simulink model "Parabolic_alpha_sim"  (R2017a)
settings: Solver=FixedStepAuto  StartTime=0.0  StopTime=4  FixedStep=2e-4  RelTol=1e-3
values from neighbouring files (symbols this model uses):
  b = 2.8956    [Aerosonde_coeff.m]    (also in coeff_Aerosonde.m)
  c = 0.18994    [Aerosonde_coeff.m]    (also in coeff_Aerosonde.m)
  C_De = 0    [Aerosonde_coeff.m]    (also in coeff_Aerosonde.m)
  C_Dl_quad = 0.05*2    (= 0.1)    [coeff_quad.m]    (also in init_quad.m = 0.05)
  C_Dq = 0    [Aerosonde_coeff.m]    (also in coeff_Aerosonde.m)
  C_Dq_quad = 0.5    [coeff_quad.m]    (also in init_quad.m)
  C_Le = -0.36    [Aerosonde_coeff.m]    (also in coeff_Aerosonde.m)
  C_Lq = 0    [Aerosonde_coeff.m]    (also in coeff_Aerosonde.m)
  C_m0 = -0.02338    [Aerosonde_coeff.m]    (also in coeff_Aerosonde.m)
  C_ma = -0.38    [Aerosonde_coeff.m]    (also in coeff_Aerosonde.m)
  C_me = -0.5    [Aerosonde_coeff.m]    (also in coeff_Aerosonde.m)
  C_mq = -3.6    [Aerosonde_coeff.m]    (also in coeff_Aerosonde.m)
  d_m_quad = 0.15    [coeff_quad.m]    (also in init_quad.m)
  g = 9.81    [coeff_quad.m]    (also in init_quad.m)
  J_quad = 0.2    [coeff_quad.m]    (also in init_quad.m)
  m_quad = 2.5    [coeff_quad.m]    (also in init_quad.m)
  max_sum_force = 80    [coeff_quad.m]    (also in init_quad.m = 100)
  quad_init_theta = -20*deg2rad    [init__Aerosonde_and_quad.m]    (also in init_quad.m = -0.349065850399)
  quad_init_vx = 15    [init__Aerosonde_and_quad.m]    (also in init_quad.m)
  quad_init_vz = 0    [init__Aerosonde_and_quad.m]    (also in init_quad.m)
  quad_init_x = -8    [init__Aerosonde_and_quad.m]    (also in init_quad.m)
  quad_init_z = -dist_z-2    [init__Aerosonde_and_quad.m]    (also in init_quad.m = -20)
  rho = 1.2682    [Aerosonde_coeff.m]    (also in coeff_Aerosonde.m)
undefined symbols (not defined in the file or in its folder): Newton, Raphson
libraries: simulink_extras x8, aerolibasang x3, shared3dof x1, aerolibadyn x1
settings Model: Creator=jljoberg  LastModifiedBy=jljoberg

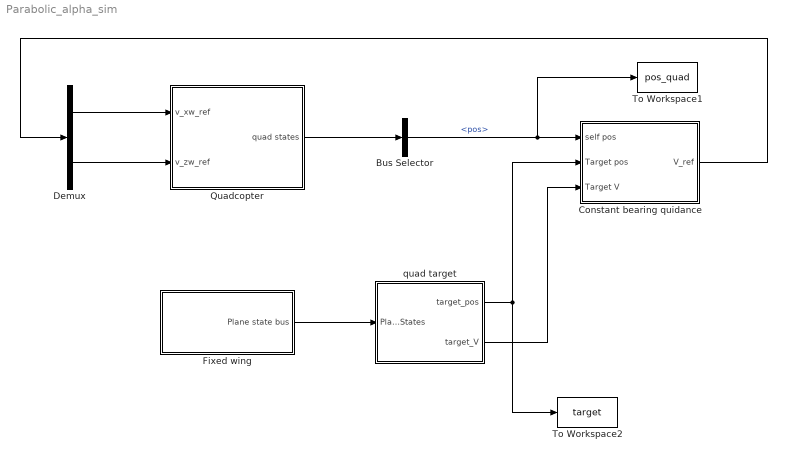
== system Parabolic_alpha_sim ==
  Bus Selector : BusSelector  OutputSignals=pos
  Constant bearing quidance : Subsystem
  Demux : Demux  Outputs=2
  Fixed wing : Subsystem
  Quadcopter : Subsystem
  To Workspace1 : ToWorkspace  VariableName=pos_quad  SaveFormat=Timeseries  SampleTime=-1
  To Workspace2 : ToWorkspace  VariableName=target  SaveFormat=Timeseries  SampleTime=-1
  quad target : Subsystem
  wires:
  Fixed wing/1(Plane state bus) -> quad target/1(Plane States)
  quad target/1(target_pos) -> Constant bearing quidance/2(Target pos), To Workspace2/1
  quad target/2(target_V) -> Constant bearing quidance/3(Target V)
  Quadcopter/1(quad states) -> Bus Selector/1
  Bus Selector/1 -> To Workspace1/1, Constant bearing quidance/1(self pos)  "<pos>"
  Constant bearing quidance/1(V_ref) -> Demux/1
  Demux/2 -> Quadcopter/2(v_zw_ref)
  Demux/1 -> Quadcopter/1(v_xw_ref)

== system Parabolic_alpha_sim/Constant bearing quidance ==
  self pos : Inport
  Target pos : Inport  Port=2
  Target V : Inport  Port=3
  CBG : MATLAB Function  TreatAsAtomicUnit=on
  V_ref : Outport
  wires:
  self pos/1 -> CBG/1(p)
  Target pos/1 -> CBG/2(p_t)
  Target V/1 -> CBG/3(V_t)
  CBG/1(V_ref) -> V_ref/1

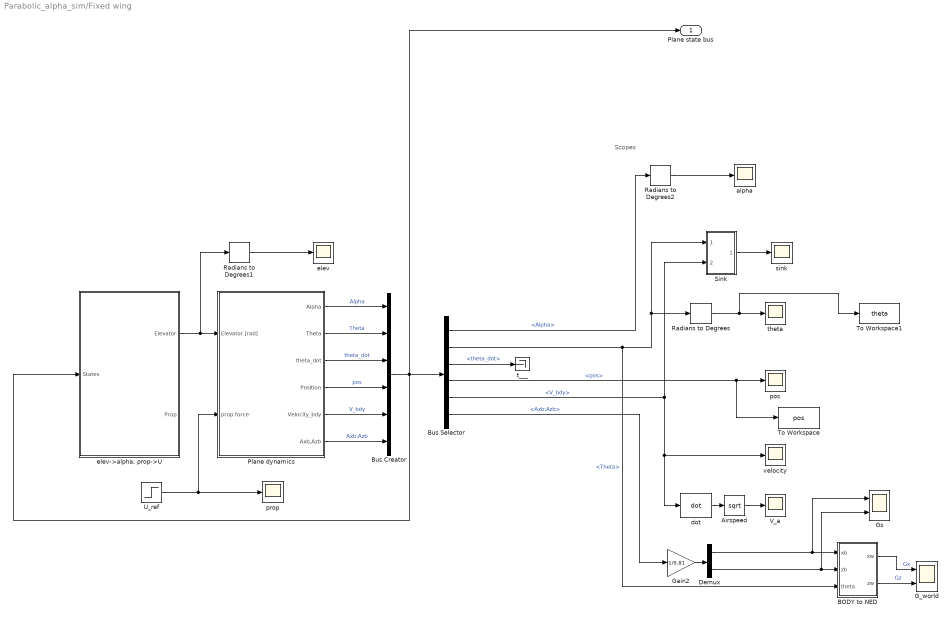
== system Parabolic_alpha_sim/Fixed wing ==
  note: Scopes
  Airspeed : Sqrt  AlgorithmType=Newton-Raphson  SaturateOnIntegerOverflow=on
  BODY to NED : Subsystem
  Bus Creator : BusCreator  Inputs=6
  Bus Selector : BusSelector  OutputSignals=Alpha,Theta,theta_dot,pos,V_bdy,Axb;Azb
  Demux : Demux  Outputs=2
  G_world : Scope  NumInputPorts=2
  Gain2 : Gain  Gain=1/9.81
  Gs : Scope  NumInputPorts=2
  Plane dynamics : Subsystem
  Radians to Degrees : simulink_extras/Transformations/Radians to Degrees
  Radians to Degrees1 : simulink_extras/Transformations/Radians to Degrees
  Radians to Degrees2 : simulink_extras/Transformations/Radians to Degrees
  Sink : Subsystem
  To Workspace : ToWorkspace  VariableName=pos  SaveFormat=Timeseries  SampleTime=-1
  To Workspace1 : ToWorkspace  VariableName=theta  SaveFormat=Timeseries  SampleTime=-1
  U_ref : Step  Time=10.5  After=0  SampleTime=0
  V_a : Scope
  alpha : Scope
  dot : aerolibasang/Incidence  & Airspeed/dot
      settings: SourceProductName=Aerospace Blockset  SourceProductBaseCode=AE
  elev : Scope
  elev->alpha; prop->U : Subsystem  VariantControl=Variant
  pos : Scope
  prop : Scope
  sink : Scope
  t___ : Terminator
  theta : Scope
  velocity : Scope
  Plane state bus : Outport
  wires:
  Plane dynamics/3(theta_dot) -> Bus Creator/3  "theta_dot"
  Plane dynamics/2(Theta) -> Bus Creator/2  "Theta"
  Plane dynamics/1(Alpha) -> Bus Creator/1  "Alpha"
  Airspeed/1 -> V_a/1
  Bus Selector/3 -> t___/1  "<theta_dot>"
  Bus Selector/4 -> To Workspace/1, pos/1  "<pos>"
  Bus Selector/5 -> dot/1, velocity/1, Sink/2(v_bdy)  "<V_bdy>"
  Bus Selector/2 -> BODY to NED/3(theta), Radians to Degrees/1, Sink/1(theta)  "<Theta>"
  Radians to Degrees/1 -> To Workspace1/1, theta/1
  Sink/1(sink) -> sink/1
  Bus Selector/1 -> Radians to Degrees2/1  "<Alpha>"
  Plane dynamics/6(Axb,Azb) -> Bus Creator/6  "Axb;Azb"
  dot/1 -> Airspeed/1
  Plane dynamics/5(Velocity_bdy) -> Bus Creator/5  "V_bdy"
  Plane dynamics/4(Position) -> Bus Creator/4  "pos"
  Demux/1 -> BODY to NED/1(xb), Gs/1
  Radians to Degrees1/1 -> elev/1
  Gain2/1 -> Demux/1
  elev->alpha; prop->U/1(Elevator) -> Radians to Degrees1/1, Plane dynamics/1(Elevator [rad])
  Demux/2 -> BODY to NED/2(zb), Gs/2
  BODY to NED/1(xw) -> G_world/1  "Gx"
  BODY to NED/2(zw) -> G_world/2  "Gz"
  Radians to Degrees2/1 -> alpha/1
  Bus Selector/6 -> Gain2/1  "<Axb;Azb>"
  U_ref/1 -> prop/1, Plane dynamics/2(prop force)
  Bus Creator/1 -> Plane state bus/1, elev->alpha; prop->U/1(States), Bus Selector/1

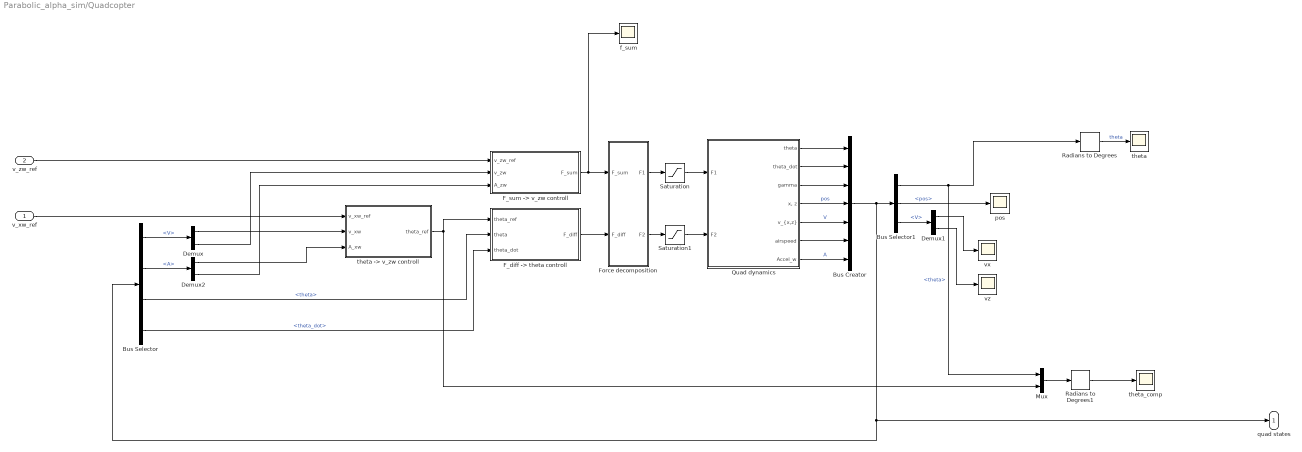
== system Parabolic_alpha_sim/Quadcopter ==
  v_xw_ref : Inport
  v_zw_ref : Inport  Port=2
  Bus Creator : BusCreator  Inputs=7
  Bus Selector : BusSelector  OutputSignals=V,A,theta,theta_dot
  Bus Selector1 : BusSelector  OutputSignals=theta,pos,V
  Demux : Demux  Outputs=2
  Demux1 : Demux  Outputs=2
  Demux2 : Demux  Outputs=2
  "F_diff -> theta controll" : Subsystem
  "F_sum -> v_zw controll" : Subsystem
  Force decomposition : Subsystem
  Mux : Mux  Inputs=2
  Quad dynamics : Subsystem
  Radians to Degrees : simulink_extras/Transformations/Radians to Degrees
  Radians to Degrees1 : simulink_extras/Transformations/Radians to Degrees
  Saturation : Saturate  UpperLimit=max_sum_force/2  LowerLimit=-max_sum_force/2
  Saturation1 : Saturate  UpperLimit=max_sum_force/2  LowerLimit=-max_sum_force/2
  f_sum : Scope
  "pos " : Scope
  theta : Scope
  "theta -> v_zw controll" : Subsystem
  theta_comp : Scope
  vx : Scope
  "vz " : Scope
  quad states : Outport
  wires:
  Force decomposition/2(F2) -> Saturation1/1
  Bus Selector/4 -> "F_diff -> theta controll"/3(theta_dot)  "<theta_dot>"
  Bus Selector/3 -> "F_diff -> theta controll"/2(theta)  "<theta>"
  Quad dynamics/7(Accel_w) -> Bus Creator/7  "A"
  Saturation1/1 -> Quad dynamics/2(F2)
  Saturation/1 -> Quad dynamics/1(F1)
  Radians to Degrees/1 -> theta/1  "theta"
  Demux1/2 -> "vz "/1
  Quad dynamics/6(airspeed) -> Bus Creator/6
  v_zw_ref/1 -> "F_sum -> v_zw controll"/1(v_zw_ref)
  "F_sum -> v_zw controll"/1(F_sum) -> f_sum/1, Force decomposition/1(F_sum)
  Bus Creator/1 -> Bus Selector/1, quad states/1, Bus Selector1/1
  Bus Selector/1 -> Demux/1  "<V>"
  Quad dynamics/2(theta_dot) -> Bus Creator/2
  Bus Selector/2 -> Demux2/1  "<A>"
  Demux/1 -> "theta -> v_zw controll"/2(v_xw)
  Demux2/1 -> "theta -> v_zw controll"/3(A_xw)
  Bus Selector1/2 -> "pos "/1  "<pos>"
  Quad dynamics/3(gamma) -> Bus Creator/3
  Quad dynamics/4("x, z") -> Bus Creator/4  "pos"
  Bus Selector1/3 -> Demux1/1  "<V>"
  Quad dynamics/1(theta) -> Bus Creator/1
  Radians to Degrees1/1 -> theta_comp/1
  Quad dynamics/5("v_{x,z}") -> Bus Creator/5  "V"
  Bus Selector1/1 -> Mux/1, Radians to Degrees/1  "<theta>"
  Demux/2 -> "F_sum -> v_zw controll"/2(v_zw)
  "theta -> v_zw controll"/1(theta_ref) -> Mux/2, "F_diff -> theta controll"/1(theta_ref)
  Force decomposition/1(F1) -> Saturation/1
  Mux/1 -> Radians to Degrees1/1
  Demux2/2 -> "F_sum -> v_zw controll"/3(A_zw)
  Demux1/1 -> vx/1
  "F_diff -> theta controll"/1(F_diff) -> Force decomposition/2(F_diff)
  v_xw_ref/1 -> "theta -> v_zw controll"/1(v_xw_ref)

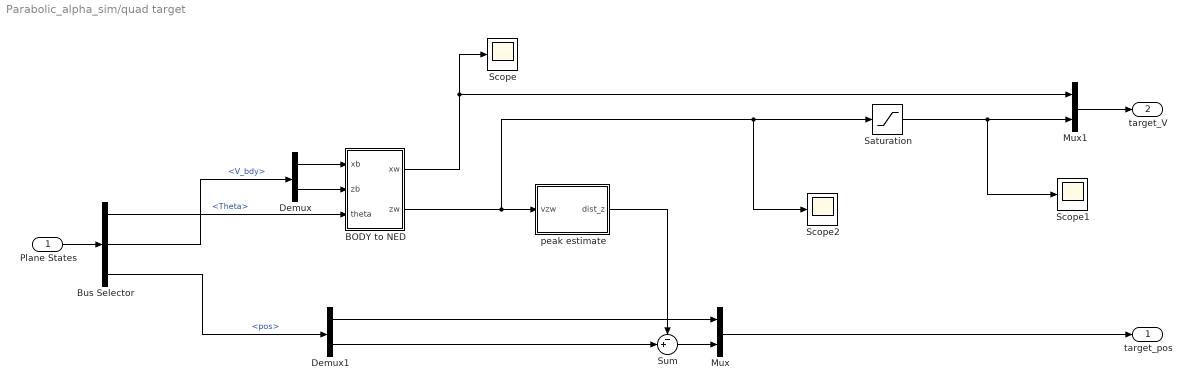
== system Parabolic_alpha_sim/quad target ==
  Plane States : Inport
  BODY to NED : Subsystem
  Bus Selector : BusSelector  OutputSignals=Theta,V_bdy,pos
  Demux : Demux  Outputs=2
  Demux1 : Demux  Outputs=2
  Mux : Mux  Inputs=2
  Mux1 : Mux  Inputs=2
  Saturation : Saturate  UpperLimit=inf  LowerLimit=0
  Scope : Scope
  Scope1 : Scope
  Scope2 : Scope
  Sum : Sum  Inputs=-+|
  peak estimate : MATLAB Function  TreatAsAtomicUnit=on
  target_pos : Outport
  target_V : Outport  Port=2
  wires:
  Plane States/1 -> Bus Selector/1
  Bus Selector/2 -> Demux/1  "<V_bdy>"
  Bus Selector/1 -> BODY to NED/3(theta)  "<Theta>"
  Demux/1 -> BODY to NED/1(xb)
  Demux/2 -> BODY to NED/2(zb)
  Bus Selector/3 -> Demux1/1  "<pos>"
  BODY to NED/2(zw) -> Scope2/1, Saturation/1, peak estimate/1(vzw)
  Demux1/2 -> Sum/2
  Demux1/1 -> Mux/1
  Sum/1 -> Mux/2
  Mux/1 -> target_pos/1
  BODY to NED/1(xw) -> Mux1/1, Scope/1
  Mux1/1 -> target_V/1
  peak estimate/1(dist_z) -> Sum/1
  Saturation/1 -> Scope1/1, Mux1/2

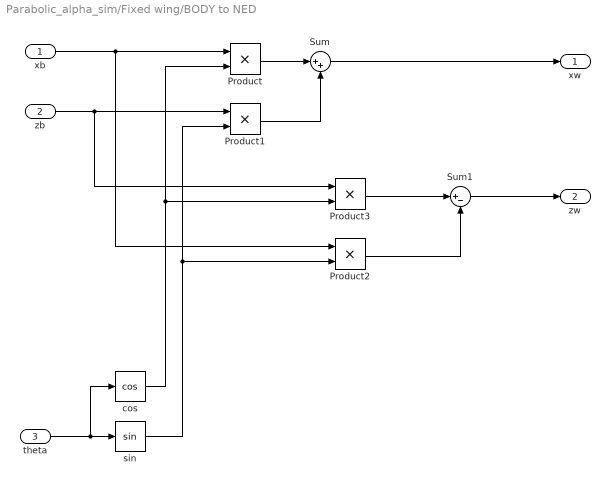
== system Parabolic_alpha_sim/Fixed wing/BODY to NED ==
  xb : Inport
  zb : Inport  Port=2
  theta : Inport  Port=3
  Product{,1..3} (4 alike) : Product
  Sum : Sum  Inputs=|++
  Sum1 : Sum  Inputs=|+-
  "cos " : Trigonometry  Operator=cos
  sin : Trigonometry
  xw : Outport
  zw : Outport  Port=2
  wires:
  theta/1 -> sin/1, "cos "/1
  xb/1 -> Product/1, Product2/1
  "cos "/1 -> Product3/2, Product/2
  Product/1 -> Sum/1
  Sum/1 -> xw/1
  zb/1 -> Product3/1, Product1/1
  sin/1 -> Product1/2, Product2/2
  Product1/1 -> Sum/2
  Sum1/1 -> zw/1
  Product3/1 -> Sum1/1
  Product2/1 -> Sum1/2

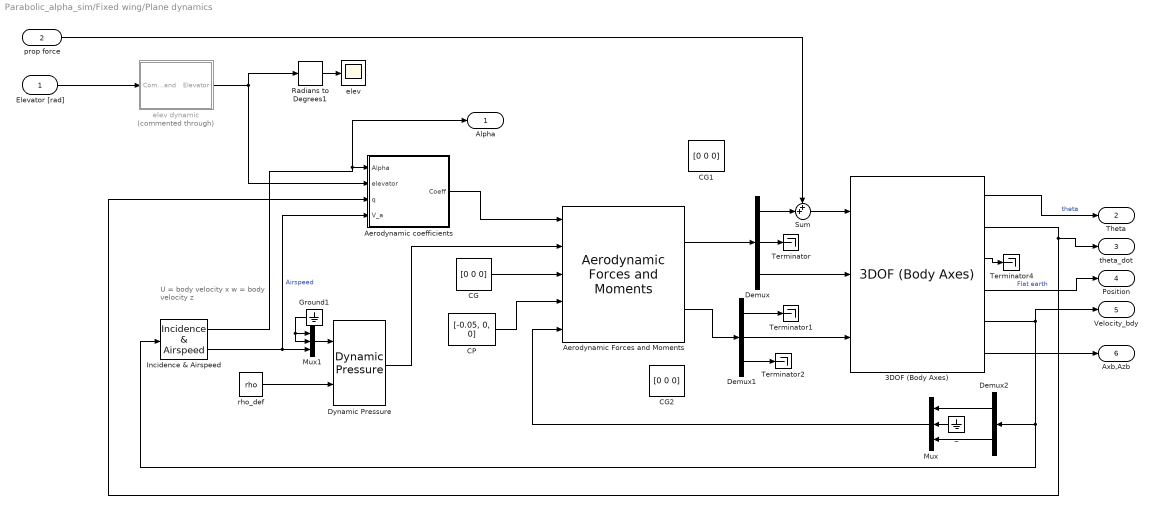
== system Parabolic_alpha_sim/Fixed wing/Plane dynamics ==
  note: U = body velocity x
      | w = body velocity z
  Elevator [rad] : Inport
  prop force : Inport  Port=2
  3DOF (Body Axes) : shared3dof/3DOF (Body Axes)  units=Metric (MKS)  mtype=Fixed  v_ini=20  theta_ini=65*deg2rad  alpha_ini=2*deg2rad  q_ini=0*deg2rad  pos_ini=[0 0]  mass=m  mass_e=0.5  mass_f=3.0  Iyy=Jy  Iyy_e=0.5  Iyy_f=3.0  g_in=Internal  g=9.81  vre_flag=on  abi_flag=off
  "Aerodynamic Forces and Moments " : aerolibadyn/Aerodynamic Forces and Moments   inputAxes=Wind  outputForceAxes=Body  outputMomentAxes=Wind  S=S  b=b  cbar=1
      settings: SourceProductName=Aerospace Blockset
  Aerodynamic coefficients : Subsystem
  CG : Constant  Value=[0 0 0]
  CG1 : Constant  Value=[0 0 0]
  CG2 : Constant  Value=[0 0 0]
  CP : Constant  Value=[-0.05, 0, 0]
  Demux : Demux  Outputs=3
  Demux1 : Demux  Outputs=3
  Demux2 : Demux  Outputs=2
  Dynamic Pressure : aerolibasang/Dynamic Pressure
  Ground1 : Ground
  Incidence & Airspeed : aerolibasang/Incidence  & Airspeed
      settings: SourceProductName=Aerospace Blockset  SourceProductBaseCode=AE
  Mux : Mux  Inputs=3
  Mux1 : Mux  Inputs=3
  Radians to Degrees1 : simulink_extras/Transformations/Radians to Degrees
  Sum : Sum  Inputs=++|
  Terminator{,1..2,4} (4 alike) : Terminator
  _ : Ground
  elev : Scope
  elev dynamic : Subsystem  Commented=through
  rho_def : Constant  Value=rho
  Alpha : Outport
  Theta : Outport  Port=2
  theta_dot : Outport  Port=3
  Position : Outport  Port=4
  Velocity_bdy : Outport  Port=5
  Axb,Azb : Outport  Port=6
  wires:
  Ground1/1 -> Mux1/1, Mux1/2
  3DOF (Body Axes)/2 -> Aerodynamic coefficients/3(q), theta_dot/1
  3DOF (Body Axes)/3 -> Terminator4/1
  Incidence & Airspeed/1 -> Alpha/1, Aerodynamic coefficients/1(Alpha)
  rho_def/1 -> Dynamic Pressure/2
  Aerodynamic coefficients/1(Coeff) -> "Aerodynamic Forces and Moments "/1
  Incidence & Airspeed/2 -> Mux1/3, Aerodynamic coefficients/4(V_a)  "Airspeed"
  3DOF (Body Axes)/5 -> Velocity_bdy/1, Incidence & Airspeed/1, Demux2/1
  Dynamic Pressure/1 -> "Aerodynamic Forces and Moments "/2
  Demux/3 -> 3DOF (Body Axes)/2
  3DOF (Body Axes)/1 -> Theta/1  "theta"
  3DOF (Body Axes)/6 -> Axb,Azb/1
  Demux/2 -> Terminator/1
  3DOF (Body Axes)/4 -> Position/1  "Flat earth"
  CG/1 -> "Aerodynamic Forces and Moments "/3
  CP/1 -> "Aerodynamic Forces and Moments "/4
  Demux2/1 -> Mux/1
  Demux1/2 -> 3DOF (Body Axes)/3
  _/1 -> Mux/2
  Demux1/1 -> Terminator1/1
  Demux1/3 -> Terminator2/1
  Demux2/2 -> Mux/3
  Mux/1 -> "Aerodynamic Forces and Moments "/5
  Mux1/1 -> Dynamic Pressure/1
  Sum/1 -> 3DOF (Body Axes)/1
  prop force/1 -> Sum/1
  Demux/1 -> Sum/2
  Radians to Degrees1/1 -> elev/1
  Elevator [rad]/1 -> elev dynamic/1(Command)
  elev dynamic/1(Elevator) -> Aerodynamic coefficients/2(elevator), Radians to Degrees1/1
  "Aerodynamic Forces and Moments "/2 -> Demux1/1
  "Aerodynamic Forces and Moments "/1 -> Demux/1

== system Parabolic_alpha_sim/Fixed wing/Sink ==
  theta : Inport
  v_bdy : Inport  Port=2
  Demux : Demux  Outputs=2
  Product : Product
  Product1 : Product
  Sum : Sum  Inputs=-+|
  Trigonometric Function : Trigonometry  Operator=cos
  Trigonometric Function1 : Trigonometry
  sink : Outport
  wires:
  v_bdy/1 -> Demux/1
  theta/1 -> Trigonometric Function1/1, Trigonometric Function/1
  Product/1 -> Sum/2
  Product1/1 -> Sum/1
  Sum/1 -> sink/1
  Trigonometric Function/1 -> Product/2
  Demux/2 -> Product/1
  Demux/1 -> Product1/2
  Trigonometric Function1/1 -> Product1/1

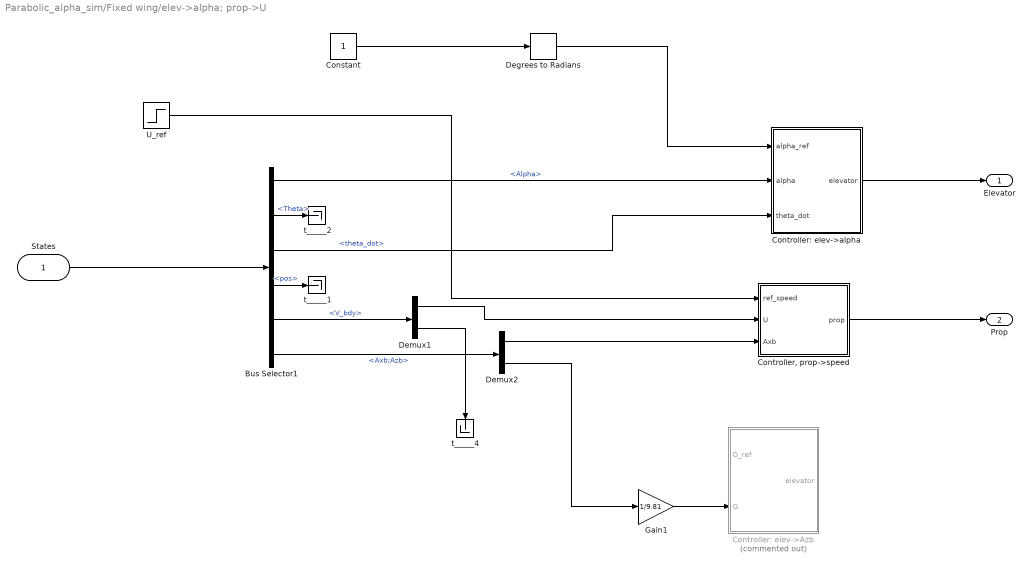
== system Parabolic_alpha_sim/Fixed wing/elev->alpha; prop->U ==
  States : Inport
  Bus Selector1 : BusSelector  OutputSignals=Alpha,Theta,theta_dot,pos,V_bdy,Axb;Azb
  Constant : Constant
  "Controller, prop->speed" : Subsystem
  Controller: elev->Azb : Subsystem  Commented=on
  Controller: elev->alpha : Subsystem
  Degrees to Radians : simulink_extras/Transformations/Degrees to Radians
  Demux1 : Demux  Outputs=2
  Demux2 : Demux  Outputs=2
  Gain1 : Gain  Gain=1/9.81
  U_ref : Step  Time=150  Before=25  After=25  SampleTime=0
  t_____1 : Terminator
  t_____2 : Terminator
  t_____4 : Terminator
  Elevator : Outport
  Prop : Outport  Port=2
  wires:
  "Controller, prop->speed"/1(prop) -> Prop/1
  Demux1/1 -> "Controller, prop->speed"/2(U)
  Demux2/2 -> Gain1/1
  Bus Selector1/5 -> Demux1/1  "<V_bdy>"
  Bus Selector1/6 -> Demux2/1  "<Axb;Azb>"
  Demux2/1 -> "Controller, prop->speed"/3(Axb)
  States/1 -> Bus Selector1/1
  Demux1/2 -> t_____4/1
  Bus Selector1/4 -> t_____1/1  "<pos>"
  Gain1/1 -> Controller: elev->Azb/2(G)
  Controller: elev->alpha/1(elevator) -> Elevator/1
  Bus Selector1/1 -> Controller: elev->alpha/2(alpha)  "<Alpha>"
  U_ref/1 -> "Controller, prop->speed"/1(ref_speed)
  Degrees to Radians/1 -> Controller: elev->alpha/1(alpha_ref)
  Bus Selector1/2 -> t_____2/1  "<Theta>"
  Bus Selector1/3 -> Controller: elev->alpha/3(theta_dot)  "<theta_dot>"
  Constant/1 -> Degrees to Radians/1

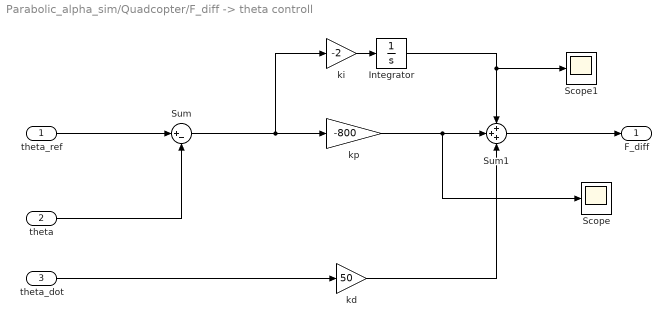
== system Parabolic_alpha_sim/Quadcopter/F_diff -> theta controll ==
  theta_ref : Inport
  theta : Inport  Port=2
  theta_dot : Inport  Port=3
  Integrator : Integrator
  Scope : Scope
  Scope1 : Scope
  Sum : Sum  Inputs=|+-
  Sum1 : Sum  Inputs=+++
  kd : Gain  Gain=50
  ki : Gain  Gain=-2
  kp : Gain  Gain=-800
  F_diff : Outport
  wires:
  kp/1 -> Scope/1, Sum1/2
  Sum1/1 -> F_diff/1
  Sum/1 -> kp/1, ki/1
  ki/1 -> Integrator/1
  theta/1 -> Sum/2
  theta_ref/1 -> Sum/1
  theta_dot/1 -> kd/1
  kd/1 -> Sum1/3
  Integrator/1 -> Scope1/1, Sum1/1

== system Parabolic_alpha_sim/Quadcopter/F_sum -> v_zw controll ==
  v_zw_ref : Inport
  v_zw : Inport  Port=2
  A_zw : Inport  Port=3
  Integrator : Integrator  LimitOutput=on  UpperSaturationLimit=max_sum_force  LowerSaturationLimit=-max_sum_force
  Saturation : Saturate  UpperLimit=max_sum_force  LowerLimit=-max_sum_force
  Scope : Scope
  Sum : Sum  Inputs=|+-
  Sum1 : Sum  Inputs=+++
  kd : Gain  Gain=4
  ki : Gain  Gain=-40
  kp : Gain  Gain=-60
  F_sum : Outport
  wires:
  v_zw_ref/1 -> Sum/1
  v_zw/1 -> Sum/2
  ki/1 -> Integrator/1
  Sum/1 -> ki/1, kp/1
  Integrator/1 -> Scope/1, Sum1/1
  Sum1/1 -> Saturation/1
  kp/1 -> Sum1/2
  A_zw/1 -> kd/1
  kd/1 -> Sum1/3
  Saturation/1 -> F_sum/1

== system Parabolic_alpha_sim/Quadcopter/Force decomposition ==
  F_sum : Inport
  F_diff : Inport  Port=2
  Gain : Gain  Gain=1/2
  Gain1 : Gain  Gain=1/2
  Sum : Sum  Inputs=|++
  Sum1 : Sum  Inputs=-+|
  F1 : Outport
  F2 : Outport  Port=2
  wires:
  Sum/1 -> F1/1
  Sum1/1 -> F2/1
  Gain/1 -> Sum1/2, Sum/1
  F_diff/1 -> Gain1/1
  Gain1/1 -> Sum1/1, Sum/2
  F_sum/1 -> Gain/1

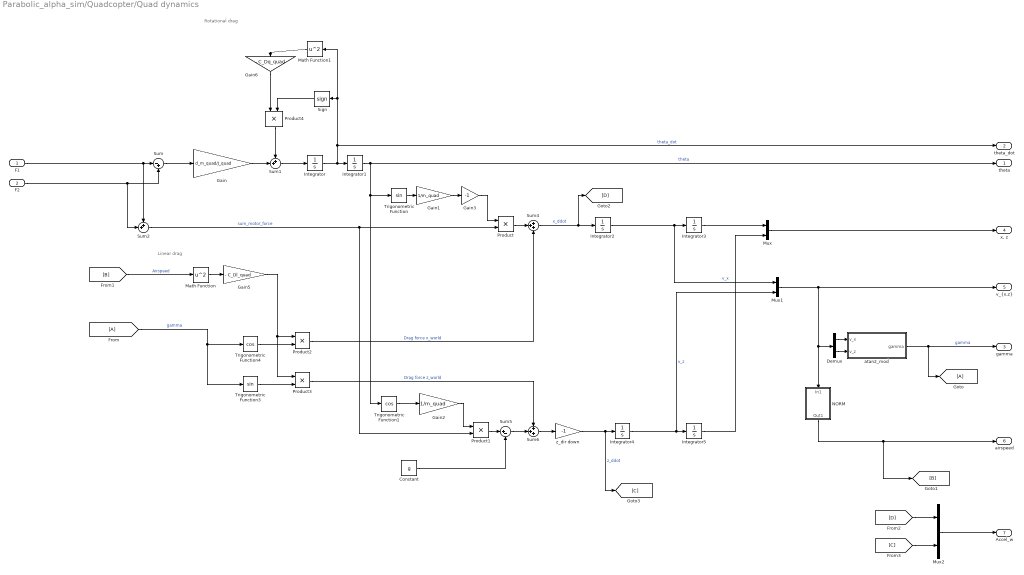
== system Parabolic_alpha_sim/Quadcopter/Quad dynamics ==
  note: Rotational drag
  note: Linear drag
  F1 : Inport
  F2 : Inport  Port=2
  Constant : Constant  Value=g
  Demux : Demux  Outputs=2
  Gain : Gain  Gain=d_m_quad/J_quad
  Gain1 : Gain  Gain=1/m_quad
  Gain2 : Gain  Gain=1/m_quad
  Gain3 : Gain  Gain=-1
  Gain5 : Gain  Gain=- C_Dl_quad
  Gain6 : Gain  Gain=- C_Dq_quad
  Integrator : Integrator
  Integrator1 : Integrator  InitialCondition=quad_init_theta
  Integrator2 : Integrator  InitialCondition=quad_init_vx
  Integrator3 : Integrator  InitialCondition=quad_init_x
  Integrator4 : Integrator  InitialCondition=quad_init_vz
  Integrator5 : Integrator  InitialCondition=quad_init_z
  Math Function : Math  Operator=square  SaturateOnIntegerOverflow=on
  Math Function1 : Math  Operator=square  SaturateOnIntegerOverflow=on
  Mux : Mux  Inputs=2
  Mux1 : Mux  Inputs=2
  Mux2 : Mux  Inputs=2
  NORM : Subsystem
  Product{,1..4} (5 alike) : Product
  Sign : Signum
  Sum : Sum  Inputs=|-+
  Sum1 : Sum  Inputs=++|
  Sum2 : Sum  Inputs=++|
  Sum4 : Sum  Inputs=+++
  Sum5 : Sum  Inputs=|+-
  Sum6 : Sum  Inputs=+++
  Trigonometric Function : Trigonometry
  Trigonometric Function1 : Trigonometry  Operator=cos
  Trigonometric Function3 : Trigonometry
  Trigonometric Function4 : Trigonometry  Operator=cos
  atan2_mod : MATLAB Function  TreatAsAtomicUnit=on
  z_dir down : Gain  Gain=-1
  theta : Outport
  theta_dot : Outport  Port=2
  gamma : Outport  Port=3
  "x, z" : Outport  Port=4
  "v_{x,z}" : Outport  Port=5
  airspeed : Outport  Port=6
  Accel_w : Outport  Port=7
  wires:
  Integrator/1 -> theta_dot/1, Sign/1, Math Function1/1, Integrator1/1  "theta_dot"
  Integrator1/1 -> Trigonometric Function1/1, Trigonometric Function/1, theta/1  "theta"
  F1/1 -> Sum2/1, Sum/1
  F2/1 -> Sum2/2, Sum/2
  Sum/1 -> Gain/1
  Gain/1 -> Sum1/2
  Sum1/1 -> Integrator/1
  Integrator2/1 -> Mux1/1, Integrator3/1  "v_x"
  Trigonometric Function/1 -> Gain1/1
  Gain1/1 -> Gain3/1
  Sum2/1 -> Product/2, Product1/2  "sum_motor_force"
  Product/1 -> Sum4/2
  Sum4/1 -> [D], Integrator2/1  "x_ddot"
  Integrator4/1 -> Mux1/2, Integrator5/1  "v_z"
  Integrator5/1 -> Mux/2
  Gain2/1 -> Product1/1
  Sum5/1 -> Sum6/2
  Sum6/1 -> z_dir down/1
  Trigonometric Function1/1 -> Gain2/1
  Mux/1 -> "x, z"/1
  Integrator3/1 -> Mux/1
  Mux1/1 -> NORM/1(In1), Demux/1, "v_{x,z}"/1
  NORM/1(Out1) -> [B], airspeed/1
  Demux/1 -> atan2_mod/1(v_x)
  Demux/2 -> atan2_mod/2(v_z)
  atan2_mod/1(gamma) -> [A], gamma/1  "gamma"
  [A] -> Trigonometric Function3/1, Trigonometric Function4/1  "gamma"
  [B] -> Math Function/1  "Airspeed"
  Math Function/1 -> Gain5/1
  Gain5/1 -> Product3/1, Product2/1
  Trigonometric Function4/1 -> Product2/2
  Trigonometric Function3/1 -> Product3/2
  Math Function1/1 -> Gain6/1
  Product3/1 -> Sum6/1  "Drag force z_world"
  Product2/1 -> Sum4/3  "Drag force x_world"
  Gain6/1 -> Product4/1
  Sign/1 -> Product4/2
  Product4/1 -> Sum1/1
  Product1/1 -> Sum5/1
  Constant/1 -> Sum5/2
  z_dir down/1 -> [C], Integrator4/1  "z_ddot"
  [C] -> Mux2/2
  [D] -> Mux2/1
  Mux2/1 -> Accel_w/1
  Gain3/1 -> Product/1

== system Parabolic_alpha_sim/Quadcopter/theta -> v_zw controll ==
  v_xw_ref : Inport
  v_xw : Inport  Port=2
  A_xw : Inport  Port=3
  Ground : Ground
  Integrator : Integrator  LimitOutput=on  UpperSaturationLimit=80*deg2rad  LowerSaturationLimit=-80*deg2rad
  Saturation : Saturate  UpperLimit=80*deg2rad  LowerLimit=-80*deg2rad
  Sum : Sum  Inputs=|+-
  Sum1 : Sum  Inputs=+++
  Terminator : Terminator
  ki : Gain  Gain=-0.07
  kp : Gain  Gain=-0.5
  theta_ref : Outport
  wires:
  kp/1 -> Sum1/2
  Sum1/1 -> Saturation/1
  Integrator/1 -> Sum1/1
  ki/1 -> Integrator/1
  v_xw/1 -> Sum/2
  v_xw_ref/1 -> Sum/1
  Saturation/1 -> theta_ref/1
  Sum/1 -> ki/1, kp/1
  A_xw/1 -> Terminator/1
  Ground/1 -> Sum1/3

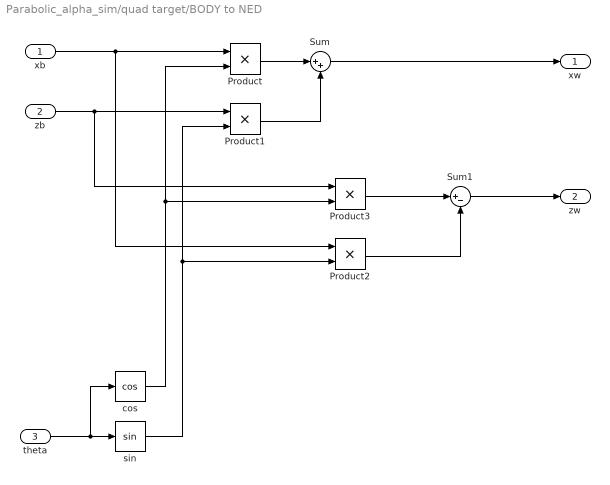
== system Parabolic_alpha_sim/quad target/BODY to NED ==
  xb : Inport
  zb : Inport  Port=2
  theta : Inport  Port=3
  Product{,1..3} (4 alike) : Product
  Sum : Sum  Inputs=|++
  Sum1 : Sum  Inputs=|+-
  "cos " : Trigonometry  Operator=cos
  sin : Trigonometry
  xw : Outport
  zw : Outport  Port=2
  wires:
  theta/1 -> sin/1, "cos "/1
  xb/1 -> Product/1, Product2/1
  "cos "/1 -> Product3/2, Product/2
  Product/1 -> Sum/1
  Sum/1 -> xw/1
  zb/1 -> Product3/1, Product1/1
  sin/1 -> Product1/2, Product2/2
  Product1/1 -> Sum/2
  Sum1/1 -> zw/1
  Product3/1 -> Sum1/1
  Product2/1 -> Sum1/2

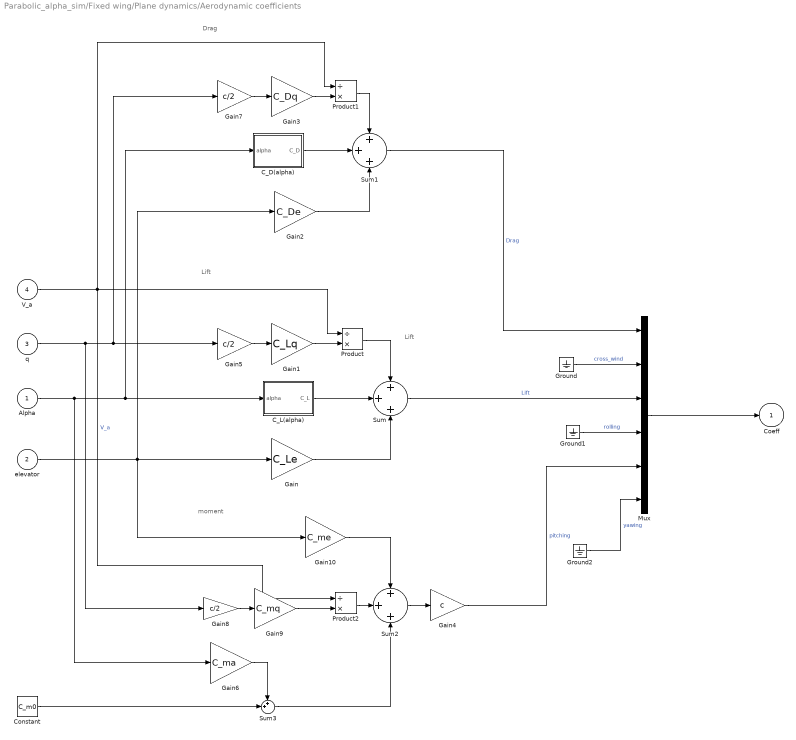
== system Parabolic_alpha_sim/Fixed wing/Plane dynamics/Aerodynamic coefficients ==
  note: moment
  note: Lift
  note: Drag
  note: Lift
  Alpha : Inport
  elevator : Inport  Port=2
  q : Inport  Port=3
  V_a : Inport  Port=4
  C_D(alpha) : MATLAB Function  TreatAsAtomicUnit=on
  C_L(alpha) : MATLAB Function  TreatAsAtomicUnit=on
  Constant : Constant  Value=C_m0
  Gain : Gain  Gain=C_Le
  Gain1 : Gain  Gain=C_Lq
  Gain10 : Gain  Gain=C_me
  Gain2 : Gain  Gain=C_De
  Gain3 : Gain  Gain=C_Dq
  Gain4 : Gain  Gain=c
  Gain5 : Gain  Gain=c/2
  Gain6 : Gain  Gain=C_ma
  Gain7 : Gain  Gain=c/2
  Gain8 : Gain  Gain=c/2
  Gain9 : Gain  Gain=C_mq
  Ground : Ground
  Ground1 : Ground
  Ground2 : Ground
  Mux : Mux  Inputs=6
  Product : Product  Inputs=/*
  Product1 : Product  Inputs=/*
  Product2 : Product  Inputs=/*
  Sum : Sum  Inputs=+++
  Sum1 : Sum  Inputs=+++
  Sum2 : Sum  Inputs=+++
  Sum3 : Sum  Inputs=++|
  Coeff : Outport
  wires:
  Alpha/1 -> Gain6/1, C_D(alpha)/1(alpha), C_L(alpha)/1(alpha)
  C_L(alpha)/1(C_L) -> Sum/2
  Gain/1 -> Sum/3
  Sum/1 -> Mux/3  "Lift"
  Ground/1 -> Mux/2  "cross_wind"
  Ground1/1 -> Mux/4  "rolling"
  Ground2/1 -> Mux/6  "yawing"
  C_D(alpha)/1(C_D) -> Sum1/2
  Gain2/1 -> Sum1/3
  q/1 -> Gain8/1, Gain7/1, Gain5/1
  V_a/1 -> Product2/1, Product/1, Product1/1  "V_a"
  Gain1/1 -> Product/2
  Product/1 -> Sum/1
  Gain5/1 -> Gain1/1
  Gain3/1 -> Product1/2
  Product1/1 -> Sum1/1
  Gain7/1 -> Gain3/1
  Sum1/1 -> Mux/1  "Drag"
  Sum2/1 -> Gain4/1
  Gain4/1 -> Mux/5  "pitching"
  Constant/1 -> Sum3/2
  Sum3/1 -> Sum2/3
  Gain6/1 -> Sum3/1
  Product2/1 -> Sum2/2
  Gain8/1 -> Gain9/1
  Gain9/1 -> Product2/2
  Gain10/1 -> Sum2/1
  elevator/1 -> Gain10/1, Gain2/1, Gain/1
  Mux/1 -> Coeff/1

== system Parabolic_alpha_sim/Fixed wing/Plane dynamics/elev dynamic ==
  Command : Inport
  Gain : Gain  Gain=9999
  Integrator : Integrator
  Scope : Scope
  Sum : Sum  Inputs=|+-
  Elevator : Outport
  wires:
  Integrator/1 -> Scope/1, Elevator/1, Sum/2
  Sum/1 -> Gain/1
  Gain/1 -> Integrator/1
  Command/1 -> Sum/1

== system Parabolic_alpha_sim/Fixed wing/elev->alpha; prop->U/Controller, prop->speed ==
  ref_speed : Inport
  U : Inport  Port=2
  Axb : Inport  Port=3
  Integrator : Integrator
  Saturation : Saturate  UpperLimit=80*1  LowerLimit=-80
  Sum : Sum  Inputs=+++
  Sum1 : Sum  Inputs=|+-
  kd : Gain  Gain=-70
  ki : Gain  Gain=0.5
  kp : Gain  Gain=20
  prop : Outport
  wires:
  Sum/1 -> Saturation/1
  kp/1 -> Sum/2
  ki/1 -> Integrator/1
  Integrator/1 -> Sum/1
  kd/1 -> Sum/3
  Axb/1 -> kd/1
  Sum1/1 -> ki/1, kp/1
  ref_speed/1 -> Sum1/1
  U/1 -> Sum1/2
  Saturation/1 -> prop/1

== system Parabolic_alpha_sim/Fixed wing/elev->alpha; prop->U/Controller: elev->Azb ==
  G_ref : Inport
  G : Inport  Port=2
  Integrator : Integrator
  Saturation : Saturate  UpperLimit=2*pi/5  LowerLimit=-2*pi/5
  Sum : Sum  Inputs=+-|
  Sum1 : Sum  Inputs=++|
  ki : Gain  Gain=-0.5
  kp : Gain  Gain=-0.1
  elevator : Outport
  wires:
  G/1 -> Sum/2
  G_ref/1 -> Sum/1
  Sum/1 -> ki/1, kp/1
  ki/1 -> Integrator/1
  kp/1 -> Sum1/2
  Integrator/1 -> Sum1/1
  Saturation/1 -> elevator/1
  Sum1/1 -> Saturation/1

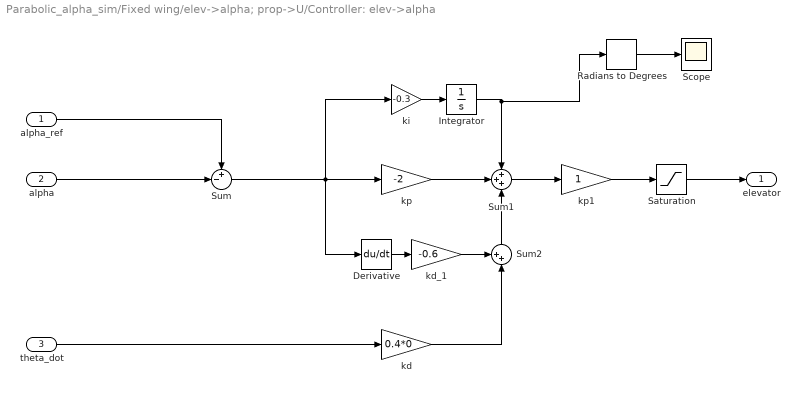
== system Parabolic_alpha_sim/Fixed wing/elev->alpha; prop->U/Controller: elev->alpha ==
  alpha_ref : Inport
  alpha : Inport  Port=2
  theta_dot : Inport  Port=3
  Derivative : Derivative
  Integrator : Integrator  InitialCondition=-5*deg2rad
  Radians to Degrees : simulink_extras/Transformations/Radians to Degrees
  Saturation : Saturate  UpperLimit=2*pi/5  LowerLimit=-2*pi/5
  Scope : Scope
  Sum : Sum  Inputs=+-|
  Sum1 : Sum  Inputs=+++
  Sum2 : Sum  Inputs=++|
  "kd " : Gain  Gain=0.4*0
  kd_1 : Gain  Gain=-0.6
  ki : Gain  Gain=-0.3
  kp : Gain  Gain=-2
  kp1 : Gain
  elevator : Outport
  wires:
  Saturation/1 -> elevator/1
  Integrator/1 -> Radians to Degrees/1, Sum1/1
  kp/1 -> Sum1/2
  ki/1 -> Integrator/1
  Sum/1 -> Derivative/1, kp/1, ki/1
  alpha_ref/1 -> Sum/1
  alpha/1 -> Sum/2
  theta_dot/1 -> "kd "/1
  Sum1/1 -> kp1/1
  Radians to Degrees/1 -> Scope/1
  Sum2/1 -> Sum1/3
  Derivative/1 -> kd_1/1
  "kd "/1 -> Sum2/2
  kd_1/1 -> Sum2/1
  kp1/1 -> Saturation/1

== system Parabolic_alpha_sim/Quadcopter/Quad dynamics/NORM ==
  In1 : Inport
  norm : MATLAB Function  TreatAsAtomicUnit=on
  Out1 : Outport
  wires:
  norm/1(V_a) -> Out1/1
  In1/1 -> norm/1(velocity)

== matlab function Parabolic_alpha_sim/Fixed wing/Plane dynamics/Aerodynamic coefficients/C_D(alpha) ==
  data: alpha input; C_D output
function C_D = C_D(alpha)


C_Dp    = 0.0437; 
C_L0    = 0.28;
C_La    = 3.45;
e       = 0.9;
S       = 0.55;
b       = 2.8956;
AR      = b^2/S;

C_D = C_Dp + (C_L0 + C_La*alpha)^2/(pi*e*AR);

== matlab function Parabolic_alpha_sim/Fixed wing/Plane dynamics/Aerodynamic coefficients/C_L(alpha) ==
  data: alpha input; C_L output
function C_L = C_L(alpha)

C_L0    = 0.28; 
C_La    = 3.45;
M       = 50;

alpha_0 = 0.4712;
sigma =( 1+exp(-M*(alpha-alpha_0))+exp(M*(alpha+alpha_0)) ) ...
              / ( (1+exp(-M*(alpha-alpha_0)))*(1+exp(M*(alpha+alpha_0))) );


C_L = (1-sigma) * (C_L0 + C_La*alpha) ...
             + sigma * 2*sign(alpha)*sin(alpha)^2*cos(alpha);

== matlab function Parabolic_alpha_sim/quad target/peak estimate ==
  data: vzw input; dist_z output
function dist_z = fcn(vzw)
    g = 9.81*0.92;
    dist_z = 1/2*vzw^2/g;
    dist_z = norm(dist_z);
    if vzw > 0.05;
        dist_z = 0;
    end
end

== matlab function Parabolic_alpha_sim/Quadcopter/Quad dynamics/NORM/norm ==
  data: velocity input; V_a output
function V_a = norm(velocity)
V_a = norm(velocity);

== matlab function Parabolic_alpha_sim/Quadcopter/Quad dynamics/atan2_mod ==
  data: v_x input; gamma output; v_z input
function gamma = atan2_mod(v_x,v_z)

if v_x == 0
    gamma = 90;
    if v_z == 0
        gamma = 0;
    end
else
    gamma = atan2(v_z,v_x);
end
gamma = -gamma;
end

== matlab function Parabolic_alpha_sim/Constant bearing quidance/CBG ==
  data: p input; V_ref output; p_t input; V_t input
function V_ref = CBG(p, p_t, V_t)

V_approach = 3*(p_t-p);

V_ref = V_approach + V_t;
